simulink model "TVCRocketSim"  (R2024b)
settings: Solver=VariableStepAuto  StartTime=0.0  StopTime=9  RelTol=1e-3
model workspace (MAT data in the model file):
  old_pitch = 0
undefined symbols (not defined in the file or in its folder): aeroData, env, q_i, thrustData, thrustTime, vehicle, x
settings Model: Creator=hroho  LastModifiedBy=Hunter Rohovit
settings SolverCC: ZeroCrossAlgorithm=Adaptive
settings DebuggingCC: MaskedZcDiagnostic=none  IgnoredZcDiagnostic=none

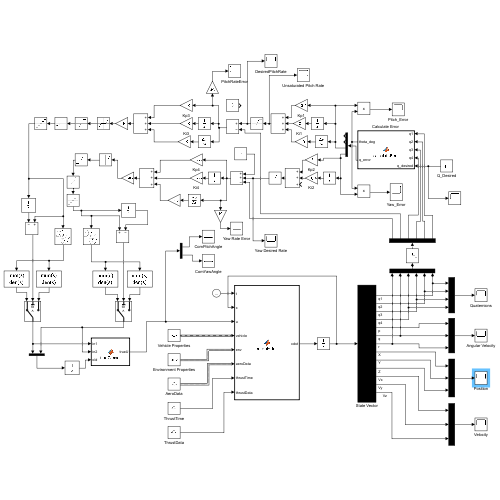
[thumbnail: Simulink's stored preview of the top-level diagram]
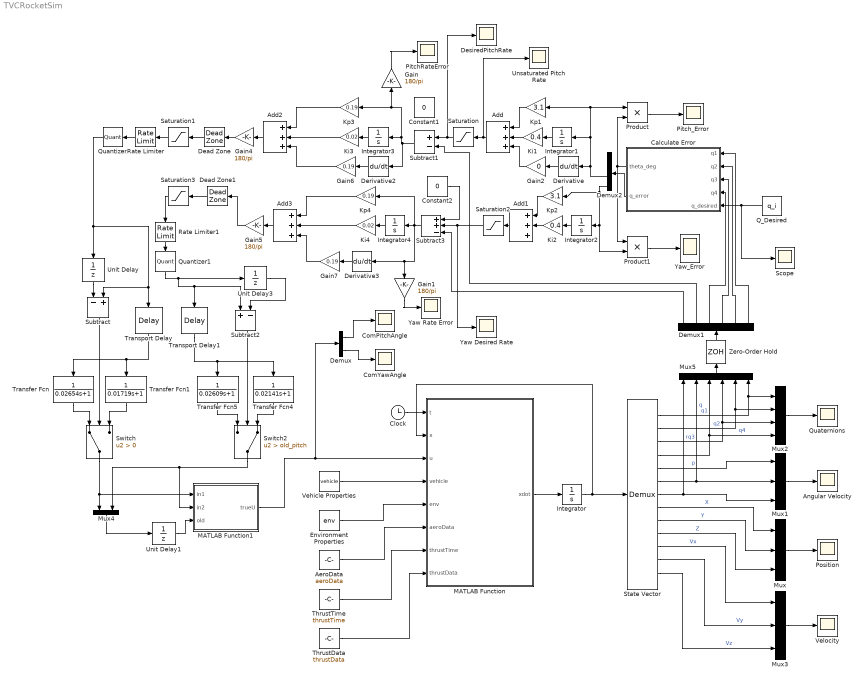
== system TVCRocketSim ==
  Add{,1..3} (4 alike) : Sum  Inputs=+++
  AeroData : Constant  Value=aeroData  OutDataTypeStr=Bus: slBus3
  Angular Velocity : Scope
  "Calculate Error " : MATLAB Function  TreatAsAtomicUnit=on
  Clock : Clock
  ComPitchAngle : Scope
  ComYawAngle : Scope
  Constant1 : Constant  Value=0
  Constant2 : Constant  Value=0
  Dead Zone : DeadZone  LowerValue=-1  UpperValue=1
  Dead Zone1 : DeadZone  LowerValue=-1  UpperValue=1
  Demux : Demux  Outputs=2
  Demux1 : Demux  Outputs=6
  Demux2 : Demux
  Derivative : Derivative
  Derivative2 : Derivative
  Derivative3 : Derivative
  DesiredPitchRate : Scope
  Environment Properties : Constant  Value=env  OutDataTypeStr=Bus: slBus2
  Gain{,1,4..5} (4 alike) : Gain  Gain=180/pi
  Gain2 : Gain  Gain=0
  Gain6 : Gain  Gain=0.19
  Gain7 : Gain  Gain=0.19
  Integrator : Integrator  InitialCondition=x
  Integrator{1..4} (4 alike) : Integrator
  Ki1 : Gain  Gain=0.4
  Ki2 : Gain  Gain=0.4
  Ki3 : Gain  Gain=0.02
  Ki4 : Gain  Gain=0.02
  Kp1 : Gain  Gain=3.1
  Kp2 : Gain  Gain=3.1
  Kp3 : Gain  Gain=0.19
  Kp4 : Gain  Gain=0.19
  MATLAB Function : MATLAB Function  TreatAsAtomicUnit=on
  MATLAB Function1 : MATLAB Function  TreatAsAtomicUnit=on
  Mux : Mux  Inputs=3
  Mux1 : Mux  Inputs=3
  Mux2 : Mux
  Mux3 : Mux  Inputs=3
  Mux4 : Mux  Inputs=2
  Mux5 : Mux  Inputs=6
  PitchRateError : Scope
  Pitch_Error : Scope
  Position : Scope
  Product : Product
  Product1 : Product
  Q_Desired : Constant  Value=q_i
  Quantizer : Quantizer  QuantizationInterval=1
  Quantizer1 : Quantizer  QuantizationInterval=1
  Quaternions : Scope
  Rate Limiter : RateLimiter  RisingSlewLimit=250  FallingSlewLimit=-250  SampleTimeMode=inherited
  Rate Limiter1 : RateLimiter  RisingSlewLimit=250  FallingSlewLimit=-250  SampleTimeMode=inherited
  Saturation : Saturate  UpperLimit=100  LowerLimit=-100
  Saturation1 : Saturate  UpperLimit=22  LowerLimit=-22
  Saturation2 : Saturate  UpperLimit=80  LowerLimit=-80
  Saturation3 : Saturate  UpperLimit=22  LowerLimit=-22
  Scope : Scope
  State Vector : Demux  Outputs=13
  Subtract : Sum  Inputs=-+
  Subtract1 : Sum  Inputs=+-
  Subtract2 : Sum  Inputs=-+
  Subtract3 : Sum  Inputs=++-
  Switch : Switch  Criteria=u2 > Threshold  SaturateOnIntegerOverflow=off  InputSameDT=off
  Switch2 : Switch  Criteria=u2 > Threshold  Threshold=old_pitch  SaturateOnIntegerOverflow=off  InputSameDT=off
  ThrustData : Constant  Value=thrustData
  ThrustTime : Constant  Value=thrustTime
  Transfer Fcn : TransferFcn  Denominator=[0.02654 1]  ContinuousStateAttributes='pu'
  Transfer Fcn1 : TransferFcn  Denominator=[0.01719 1]  ContinuousStateAttributes='pd'
  Transfer Fcn4 : TransferFcn  Denominator=[0.02141 1]  ContinuousStateAttributes='yd'
  Transfer Fcn5 : TransferFcn  Denominator=[0.02609 1]  ContinuousStateAttributes='yu'
  Transport Delay : TransportDelay  DelayTime=0.05182  BufferSize=1048576
  Transport Delay1 : TransportDelay  DelayTime=0.05182  BufferSize=1048576
  Unit Delay : UnitDelay  SampleTime=-1  HasFrameUpgradeWarning=on
  Unit Delay1 : UnitDelay  SampleTime=-1  HasFrameUpgradeWarning=on
  Unit Delay3 : UnitDelay  SampleTime=-1  HasFrameUpgradeWarning=on
  Unsaturated Pitch Rate : Scope
  Vehicle Properties : Constant  Value=vehicle  OutDataTypeStr=Bus: slBus1
  Velocity : Scope
  Yaw Desired Rate : Scope
  Yaw Rate Error : Scope
  Yaw_Error : Scope
  Zero-Order Hold : ZeroOrderHold  SampleTime=0.0025
  wires:
  MATLAB Function/1(xdot) -> Integrator/1
  Integrator/1 -> MATLAB Function/2(x), State Vector/1
  Vehicle Properties/1 -> MATLAB Function/4(vehicle)
  Environment Properties/1 -> MATLAB Function/5(env)
  AeroData/1 -> MATLAB Function/6(aeroData)
  ThrustTime/1 -> MATLAB Function/7(thrustTime)
  ThrustData/1 -> MATLAB Function/8(thrustData)
  Clock/1 -> MATLAB Function/1(t)
  Mux/1 -> Position/1
  Mux1/1 -> Angular Velocity/1
  Mux3/1 -> Velocity/1
  State Vector/13 -> Mux3/3  "Vz"
  State Vector/12 -> Mux3/2  "Vy"
  State Vector/11 -> Mux3/1  "Vx"
  State Vector/10 -> Mux/3  "Z"
  State Vector/9 -> Mux/2  "Y"
  State Vector/8 -> Mux/1  "X"
  State Vector/7 -> Mux5/6, Mux1/3  "r"
  State Vector/6 -> Mux5/5, Mux1/2  "q"
  State Vector/5 -> Mux1/1  "p"
  Mux2/1 -> Quaternions/1
  Q_Desired/1 -> Scope/1, "Calculate Error "/5(q_desired)
  Integrator1/1 -> Ki1/1
  Integrator2/1 -> Ki2/1
  Add/1 -> Unsaturated Pitch Rate/1, Saturation/1
  Kp2/1 -> Add1/1
  Kp1/1 -> Add/1
  MATLAB Function1/1(trueU) -> MATLAB Function/3(u), Demux/1
  Demux/1 -> ComPitchAngle/1
  Demux/2 -> ComYawAngle/1
  Subtract/1 -> Switch/2
  Transfer Fcn1/1 -> Switch/3
  Transfer Fcn/1 -> Switch/1
  Unit Delay/1 -> Subtract/1
  Transport Delay/1 -> Transfer Fcn/1, Transfer Fcn1/1
  Transport Delay1/1 -> Transfer Fcn4/1, Transfer Fcn5/1
  Subtract2/1 -> Switch2/2
  Transfer Fcn4/1 -> Switch2/1
  Transfer Fcn5/1 -> Switch2/3
  Unit Delay3/1 -> Subtract2/1
  Add1/1 -> Saturation2/1
  Switch2/1 -> MATLAB Function1/2(in2), Mux4/2
  Unit Delay1/1 -> MATLAB Function1/3(old)
  Mux4/1 -> Unit Delay1/1
  Ki1/1 -> Add/2
  Ki2/1 -> Add1/2
  Saturation2/1 -> Yaw Desired Rate/1, Subtract3/2
  Demux1/6 -> Subtract3/3
  Kp3/1 -> Add2/1
  Integrator3/1 -> Ki3/1
  Kp4/1 -> Add3/1
  Integrator4/1 -> Ki4/1
  Saturation1/1 -> Rate Limiter/1
  Saturation3/1 -> Rate Limiter1/1
  Zero-Order Hold/1 -> Demux1/1
  State Vector/4 -> Mux5/4, Mux2/4  "q4"
  State Vector/3 -> Mux5/3, Mux2/3  "q3"
  State Vector/2 -> Mux5/2, Mux2/2  "q2"
  State Vector/1 -> Mux5/1, Mux2/1  "q1"
  Demux1/4 -> "Calculate Error "/4(q4)
  Demux1/3 -> "Calculate Error "/3(q3)
  Demux1/2 -> "Calculate Error "/2(q2)
  Demux1/1 -> "Calculate Error "/1(q1)
  Mux5/1 -> Zero-Order Hold/1
  Quantizer/1 -> Unit Delay/1, Subtract/2, Transport Delay/1
  Quantizer1/1 -> Unit Delay3/1, Subtract2/2, Transport Delay1/1
  Rate Limiter/1 -> Quantizer/1
  Rate Limiter1/1 -> Quantizer1/1
  Switch/1 -> MATLAB Function1/1(in1), Mux4/1
  Constant2/1 -> Subtract3/1
  Saturation/1 -> Subtract1/1, DesiredPitchRate/1
  Demux1/5 -> Subtract1/2
  "Calculate Error "/2(q_error) -> Demux2/1
  Demux2/4 -> Product1/2, Integrator2/1, Kp2/1
  Demux2/3 -> Derivative/1, Product/1, Kp1/1, Integrator1/1
  Add2/1 -> Gain4/1
  Add3/1 -> Gain5/1
  Subtract1/1 -> Derivative2/1, Kp3/1, Gain/1, Integrator3/1
  Subtract3/1 -> Derivative3/1, Gain1/1, Kp4/1, Integrator4/1
  Gain5/1 -> Dead Zone1/1
  Dead Zone1/1 -> Saturation3/1
  Gain4/1 -> Dead Zone/1
  Dead Zone/1 -> Saturation1/1
  Gain/1 -> PitchRateError/1
  Gain1/1 -> Yaw Rate Error/1
  Derivative2/1 -> Gain6/1
  Gain7/1 -> Add3/3
  Derivative3/1 -> Gain7/1
  Gain6/1 -> Add2/3
  Product/1 -> Pitch_Error/1
  "Calculate Error "/1(theta_deg) -> Product/2, Product1/1
  Product1/1 -> Yaw_Error/1
  Derivative/1 -> Gain2/1
  Gain2/1 -> Add/3
  Ki3/1 -> Add2/2
  Ki4/1 -> Add3/2

== matlab function TVCRocketSim/Calculate Error  ==
  data: theta_deg output; q1 input; q2 input; q3 input; q4 input; q_error output; q_desired input
function [theta_deg, q_error] = calculateError(q1, q2, q3, q4, q_desired)
    % Compute the conjugate of the current quaternion
    q_conj = [q1, -q2, -q3, -q4];

    % Unpack components
    w1 = q_desired(1); x1 = q_desired(2); y1 = q_desired(3); z1 = q_desired(4);
    w2 = q_conj(1);    x2 = q_conj(2);    y2 = q_conj(3);    z2 = q_conj(4);

    % Manual quaternion multiplication
    w = w1*w2 - x1*x2 - y1*y2 - z1*z2;
    x = w1*x2 + x1*w2 + y1*z2 - z1*y2;
    y = w1*y2 - x1*z2 + y1*w2 + z1*x2;
    z = w1*z2 + x1*y2 - y1*x2 + z1*w2;

    % Final error quaternion
    q_error = [w, x, y, z];
    q_error = q_error / norm(q_error);  % Normalize for safety

    % Clamp to safe domain and compute angle
    w_safe = max(min(q_error(1), 1), -1);
    theta_deg = 360/pi*acos(w_safe);
end

== matlab function TVCRocketSim/MATLAB Function ==
  data: t input; x input; u input; xdot output; vehicle input; env input; aeroData input; thrustTime input; thrustData input
function xdot = rocket6dof(t,x,u,vehicle, env, aeroData, thrustTime, thrustData)
    %get values from state vector
    q = x(1:4); %quaternion components, [q0;q1;q2;q3]
    omega = x(5:7); %angular_velocity [p, q, r]
    pos = x(8:10); %position [x,y,z]
    vel = x(11:13); %velocity [Vx,Vy,Vz]

    %Quaternion kinematics matrix
    % Uses the quaternion derivative to evaluate how the quaternion changes
    % over time with angular velocity
    Omega = 0.5 * [0, -omega(1), -omega(2), -omega(3);
                  omega(1), 0, omega(3), -omega(2);
                  omega(2), -omega(3), 0, omega(1);
                  omega(3), omega(2), -omega(1), 0];

    % Compute Quaternion derivative from angular velocity
    q_dot = Omega*q;


    %create rotation matrices for transformation between vehicle 
    %and inertial reference frames 
    R_body_inertial = quat2rotm(q');
    R_inertial_body = R_body_inertial';

    %determine velocity
    v_rel_inertial = vel-env.wind(:); %velocity relative to air
    v_body = R_inertial_body * v_rel_inertial; %convert to vehicle reference frame
    v_body_mag = norm(v_body); %magnitude of free stream velocity
    if v_body_mag < 1e-6
        v_body_dir = [1; 0; 0];  % Default direction when at rest
    else
        v_body_dir = v_body / v_body_mag;
    end
    %compute total angle of attack (includes both pitch and side slip
    %angles)
    cos_theta = dot([1;0;0], v_body) / norm(v_body);
    cos_theta = max(min(cos_theta, 1), -1);  % clamp for safety
    alpha_total = acos(cos_theta); 
    alpha_total = rad2deg(alpha_total);

    alpha = atan2(v_body(3), v_body(1));  % signed AOA (Z component vs X)
    alpha = rad2deg(alpha);
    beta  = atan2(v_body(2), v_body(1));
    beta = rad2deg(beta);


    %get mass & aerodynamic properties for vehicle
    [mass, CG, I, Cd_A, Cl_A, Cy_A, ~, ~, CP, C_damp] = getVehicleProperties(t, alpha, beta, alpha_total, vehicle, aeroData); 

    %Compute Aerodynamic Forces
    q = 0.5*env.rho*v_body_mag^2; %dynamic pressure

    %drag is always in the opposite direction of velocity, paralell to the
    %rocket's longitudinal axis
    F_drag = -q*Cd_A*v_body_dir;

    %Lift is perpendicular to the velocity vector, however because this is
    %a 3d space there's an entire plane perpendicular to the velocity
    %vector. If we use a reference axis (the rocket's Z axis) we can define
    %a vector for lift
    z_body = [0;0;1]; 
    %double cross product to project z axis into the plane perpendicular to
    %the velocity vector
    lift_dir = cross(cross(v_body_dir,z_body), v_body_dir);
    lift_norm = norm(lift_dir);
    if lift_norm < 1e-6
        lift_dir = [0; 0; 0];
    else
        lift_dir = lift_dir / lift_norm;
    end
    
    F_lift = q * Cl_A * lift_dir;

    %compute the side slip force
    slip_dir = cross(-v_body_dir, lift_dir);
    slip_norm = norm(slip_dir);

    if slip_norm < 1e-6
        slip_dir = [0; 0; 0];
    else
        slip_dir = slip_dir / slip_norm;
    end

    F_slip = q * Cy_A * slip_dir;


    %Summing the forces
    F_aero_body = F_drag + F_lift + F_slip; 

    %Find force from thrust vectoring
    thrust_angle_pitch = deg2rad(u(1));
    thrust_angle_yaw = deg2rad(u(2));
    thrust_dir_body = [cos(thrust_angle_pitch)*cos(thrust_angle_yaw); sin(thrust_angle_yaw); sin(thrust_angle_pitch)];
    thrust_dir_body = thrust_dir_body/norm(thrust_dir_body);
    thrust = interp1(thrustTime(:,1), thrustData(:,1), t, 'linear', 0);
    F_thrust = thrust*thrust_dir_body;

    %Gravity Force
    F_gravity = [0;0;-env.g*mass];

    Forces_Body_Sum = F_aero_body + F_thrust; %Sum of forces in body frame of reference
    Forces_Inertial_Sum = R_body_inertial*Forces_Body_Sum + F_gravity; %Convert to inertial reference frame


    %Compute Aerodynamic Moment
    r_aero = [CG-CP;0;0]; %lever arm goes from CG to CP (+bodyX direction)
    M_aero_body = cross(r_aero, F_aero_body);

    %calculate the moments due to thrust vectoring
    %Lever arm is along the longitudinal axis of the rocket
    leverArm_pitch = [CG-vehicle.servoPitchPivotDistance; 0; 0];
    leverArm_yaw = [CG-vehicle.servoYawPivotDistance - CG; 0; 0];
    %moment = rxF
    M_pitch_thrust = cross(leverArm_pitch, F_thrust);
    M_yaw_thrust = cross(leverArm_yaw, F_thrust);
    M_thrust_body = M_yaw_thrust + M_pitch_thrust;

    %compute Aerodynamic Damping Moment
    C2A = C_damp*v_body_mag;
    M_damp = [0;-C2A*omega(2);-C2A*omega(3)];

    %Sum of moments
    Moments_Body_Sum = M_aero_body + M_thrust_body +M_damp;

    %Find the Translational Acceleration
    translational_accel = Forces_Inertial_Sum/mass;

    %Find Angular Acceleration using Euler's Equations
    angular_accel = I\(Moments_Body_Sum-cross(omega, (I*omega)));
    
    %final state derivative vector:
    xdot = [q_dot(:);
            angular_accel(:);
            vel(:);
            translational_accel(:)];
end

== matlab function TVCRocketSim/MATLAB Function1 ==
  data: in1 input; trueU output; in2 input; old input
function trueU = trueGimbal(in1, in2, old)
%%Polynomial Constants for Pitch: Found experimentally
pitchUpConstants = [7.811187e-9, -3.01114385e-7, 1.479107914e-6, 6.8529599505e-5, -0.000845657124395, 0.221847190626098, -0.706012853657809];
pitchDownConstants = [4.028134e-9, -2.13823090e-7, -9.989092799e-6, -2.1154040683e-5, 0.001950715262272, 0.241387236546681, 1.226679512304393];

%%Polynomial Constants for Yaw: Found experimentally
yawUpConstants = [-1.0287811e-8, 2.16036084e-7, 3.43473319e-7, -1.689343515e-5, 0.000217421300334, -0.242767521833985, 0.581279061853725];
yawDownConstants = [9.738129e-9, 3.29672653e-7, 2.39962733e-7, -4.9198072653e-5, -0.000602646843026, -0.250136380714918, -1.457193330894174];

if in1>old(1)
    truePitch = polyval(pitchUpConstants, in1);
else
    truePitch = polyval(pitchDownConstants, in1);
end
if in2>old(2)
    trueYaw = polyval(yawUpConstants, in2);
else
    trueYaw = polyval(yawDownConstants, in2);
end

%add in noise for the servo position
%very likely that the true servo position will not be exactly what the 
%polynomial outputs
pitchNoise = 0;%0.3*randn();
yawNoise = 0;%0.3*randn();

trueU = [truePitch+pitchNoise; trueYaw+yawNoise];
     
end
